simulink model "Autopilot_q_full_5may_new1"  (R2020a)
settings: Solver=ode4  StartTime=0.0  StopTime=300  FixedStep=0.01  RelTol=1e-3
undefined symbols (not defined in the file or in its folder): Aero_cofficients, Atmosphere_pert, Atmospheric_model, Counter_sensor_model, Earth, error_global, flags_global, Guidance_Flags_global, INT_global, param_guidance, Payload_data, Plane_state_mode_finish_catcher_ftr_mode, Plane_state_mode_finish_catcher_fw_mode, Plane_state_mode_finish_catcher_q_mode, Plane_state_mode_finish_catcher_rtr_mode, Plane_state_store, propulsion_model, propulsion_model_int, Structural_data, Thrust_data_store, time_global, WGS84, Wind_data, Wind_model_int, Wind_pert_factor
libraries: simulink x33, aerolibactuator x15, cstblocks x3, aerolibatmos2 x2, aerolibfltsims x1, aerolibtransform2 x1, shared6dof x1
(part 10 of 10)

== matlab function Autopilot_q_full_5may_new1/AUTOPILOT /Autopilot Transition mode/Reverse transition/Pitch Controller/theta controller/MATLAB Function3 ==
  data: t input; TT input; mass input; a_x_d input; theta_d output; data input
function theta_d  = fcn(t, TT, mass, a_x_d, data)
TT=sum(TT);
if (abs(TT)<1)
    TT=1;
end


while (abs(mass*a_x_d/TT)) >= 0.7 %% 45 deg max
    TT=TT+1;
end
theta_d=asin(-(mass/TT)*a_x_d);

if abs(theta_d)>20/57.3
    theta_d = sign(theta_d)*20.0/57.3;
end

end

== matlab function Autopilot_q_full_5may_new1/Plotter/ten_power_neg_5_zerorer/MATLAB Function ==
  data: u input; y output
function y = fcn(u)


for i=1:max(size(u))
    
    if (abs(u(i))<=0.000005)
        u(i)=0.0;
    end
    
end
y = u;

== matlab function Autopilot_q_full_5may_new1/Plotter/ten_power_neg_5_zerorer1/MATLAB Function ==
  data: u input; y output
function y = fcn(u)


for i=1:max(size(u))
    
    if (abs(u(i))<=0.000005)
        u(i)=0.0;
    end
    
end
y = u;

== matlab function Autopilot_q_full_5may_new1/Plotter/ten_power_neg_5_zerorer2/MATLAB Function ==
  data: u input; y output
function y = fcn(u)


for i=1:max(size(u))
    
    if (abs(u(i))<=0.000005)
        u(i)=0.0;
    end
    
end
y = u;

== matlab function Autopilot_q_full_5may_new1/Plotter/ten_power_neg_5_zerorer3/MATLAB Function ==
  data: u input; y output
function y = fcn(u)


for i=1:max(size(u))
    
    if (abs(u(i))<=0.0005)
        u(i)=0.0;
    end
    
end
y = u;

== matlab function Autopilot_q_full_5may_new1/Plotter/thrust to rpm/MATLAB Function ==
  data: motor_para input; u input; omega output; density input
function omega = fcn(motor_para, u,density)

b1=motor_para(1)*(density/1.225);
%d1=motor_para(2)*(density/1.225);

omega=(60.0/2*pi)*(sqrt(u/b1));


end

== matlab function Autopilot_q_full_5may_new1/Payload force and moment/Changing Mass/MATLAB Function ==
  data: ideal_Plane_state input; mass output
function mass = fcn(ideal_Plane_state)

Z=ideal_Plane_state(12);

if Z > 0.01
    
    Z=0.0;
    
end
if Z<-100
    Z=-100;
end
Z=abs(Z);
Z=0.0;
mass = 5 + 0.2*Z;
mass=5.0;
end

== matlab function Autopilot_q_full_5may_new1/Payload force and moment/MATLAB Function ==
  data: ideal_Plane_state input; Wind_f_m output; Wind_ned input; propulsion_data input; atmos_data input; payload_data input
function Wind_f_m = fcn(ideal_Plane_state, Wind_ned,propulsion_data,atmos_data, payload_data)

Wind_f_m = [0;0;0;0;0;0];
%%
b1=propulsion_data(1); % b and d of vtol propellers
d1=propulsion_data(2);
%%
rho=atmos_data(4); % density


if payload_data(1)==0
    
    Wind_f_m(:,:)=0.0;
    
else
u=ideal_Plane_state(1);
v=ideal_Plane_state(2);
w=ideal_Plane_state(3);
p=ideal_Plane_state(4);
q=ideal_Plane_state(5);
r=ideal_Plane_state(6);
phi=ideal_Plane_state(7);
theta=ideal_Plane_state(8);
psi=ideal_Plane_state(9);
X=ideal_Plane_state(10);
Y=ideal_Plane_state(11);
Z=ideal_Plane_state(12);

R_v_v1=[cos(psi) sin(psi) 0; -sin(psi) cos(psi) 0; 0 0 1];
R_v1_v2=[cos(theta) 0 -sin(theta) ;0 1 0; sin(theta) 0 cos(theta)];
R_v2_b=[1 0 0;0 cos(phi) sin(phi) ;0 -sin(phi) cos(phi)];
R_v_b=R_v2_b*R_v1_v2*R_v_v1;



V_wind_bd=R_v_b*[Wind_ned(1);Wind_ned(2);Wind_ned(3)];

ppp = [u-V_wind_bd(1); v-V_wind_bd(2); w-V_wind_bd(3)];
u_r=ppp(1);
v_r=ppp(2);
w_r=ppp(3);

V=sqrt(u_r^2+v_r^2+w_r^2);



if (u_r^2+v_r^2+w_r^2)<=0.001 
    alpha=0;
else
    alpha=atan2( w_r, u_r);
end


if norm(u_r) < 10^-3  && norm(v_r) < 10^-3 && norm(w_r) < 10^-3
    beta=0;
else
    beta = asin(v_r/sqrt(u_r^2+v_r^2+w_r^2));
end



R_b_s=[cos(alpha) 0 sin(alpha) ;0 1 0; -sin(alpha) 0 cos(alpha)]; 
R_s_w=[cos(beta) sin(beta) 0; -sin(beta) cos(beta) 0; 0 0 1];
R_w_b=(R_b_s)'*(R_s_w)';




if Z>0.01 
    Z=0.0;
end
    
if Z < -100
    Z = -100;
end

D = 0.5*rho*V*V*(0.2)*0.015*abs(Z);
D=0.0;
D_b=R_w_b*[-D;0;0];

Wind_f_m(1)=D_b(1);
Wind_f_m(2)=D_b(2);
Wind_f_m(3)=D_b(3);

payload_moment = D*abs(Z)/2;

p_m=R_w_b*[0;-payload_moment;0];


Wind_f_m(4)=p_m(1);
Wind_f_m(5)=p_m(2);
Wind_f_m(6)=p_m(3);


Wind_f_m(:,:)=0.0;

end
end

== matlab function Autopilot_q_full_5may_new1/Wind_Model/MATLAB Function ==
  data: L_u input; b0 output; sigma_u input; V input; a0 output; b1 output; a1 output; b2 output
function [b0,a0,b1,a1,b2]  = fcn(  L_u,sigma_u , V)

%num = sigma_u*sqrt(2*V/L_u);
%den = [1,V/L_u];

%tf_u = tf(num,den);
%%%%%%%%%%%%%%%%%%%%%%%%%%%%%%%%%%%
%% tf = b0 + b1.s + b2.s^2 ..
%%      ---------------------
%%      a0 + a1.s + a2.s^2 ..
%%%%%%%%%%%%%%%%%%%%%%%%%%%%%%%%%%%

% laplace inverse of b0/a1.s+a0  = b.e^-at
% here a0= V/L_u; b0=sigma_u*sqrt(2*V/L_u);
%a1=1;

a0= V/L_u;

b0=sigma_u*sqrt(2*V/L_u);

a1 =1;

b2=0;
b1=0;
% num=[0,0,b0];
% den=[0,a1,a0];


end

== matlab function Autopilot_q_full_5may_new1/Wind_Model/MATLAB Function1 ==
  data: t input; Alt input; L_u output; sigma_u output; light_turbulence_50 input; moderate_turbulence_50 input; light_turbulence_600 input; moderate_turbulence_600 input; L_v output; sigma_v output; L_w output; sigma_w output
function [L_u,sigma_u,L_v,sigma_v,L_w,sigma_w] = fcn(t, Alt, light_turbulence_50,moderate_turbulence_50,light_turbulence_600,moderate_turbulence_600)

L_u = 200; L_v = 200; L_w = 50;
sigma_u = 1.06; sigma_v = 1.06; sigma_w = 0.7;
L_u_lt_50 = 200;
sigma_u_lt_50 =  1.06;

L_v_lt_50 = 200;
sigma_v_lt_50 =  1.06;

L_w_lt_50 = 50;
sigma_w_lt_50 =  0.7;

L_u_mt_50 = 200;
sigma_u_mt_50 =  2.12;

L_v_mt_50 = 200;
sigma_v_mt_50 =  2.12;

L_w_mt_50 = 50;
sigma_w_mt_50 =  1.4;


L_u_lt_600 = 533;
sigma_u_lt_600 =  1.5;

L_v_lt_600 = 533;
sigma_v_lt_600 =  1.5;

L_w_lt_600 = 533;
sigma_w_lt_600 =  1.5;

L_u_mt_600 = 533;
sigma_u_mt_600 =  3.0;

L_v_mt_600 = 533;
sigma_v_mt_600 =  3.0;

L_w_mt_600 =533;
sigma_w_mt_600 =  3.0;

 Alt = -Alt;

if Alt<=50 && light_turbulence_50 ==1
    L_u = L_u_lt_50; L_v= L_v_lt_50 ; L_w = L_w_lt_50;
    sigma_u = sigma_u_lt_50; sigma_v= sigma_v_lt_50 ; sigma_w =sigma_w_lt_50;
end

if Alt<=50 && moderate_turbulence_50 == 1
    L_u = L_u_mt_50; L_v= L_v_mt_50 ; L_w = L_w_mt_50;
    sigma_u = sigma_u_mt_50; sigma_v= sigma_v_mt_50 ; sigma_w = sigma_w_mt_50;    
end

if Alt>=600 && light_turbulence_600 ==1  
    L_u = L_u_lt_600; L_v= L_v_lt_600 ; L_w = L_w_lt_600;
    sigma_u = sigma_u_lt_600; sigma_v= sigma_v_lt_600 ; sigma_w =sigma_w_lt_600;
end

if Alt>=600 && moderate_turbulence_600 == 1
    L_u = L_u_mt_600; L_v= L_v_mt_600 ; L_w = L_w_mt_600;
    sigma_u = sigma_u_mt_600; sigma_v= sigma_v_mt_600 ; sigma_w = sigma_w_mt_600;    
end

if Alt>50 && Alt<600 && light_turbulence_50 ==1 && light_turbulence_600 ==1
    L_u = (((L_u_lt_600 - L_u_lt_50)/(600-50))*(Alt-50)) + L_u_lt_50;
    L_v=L_u;
    L_w = (((L_w_lt_600 - L_w_lt_50)/(600-50))*(Alt-50)) + L_w_lt_50;
    
    sigma_u = (((sigma_u_lt_600 - sigma_u_lt_50)/(600-50))*(Alt-50)) + sigma_u_lt_50;
    sigma_v = sigma_u;
    sigma_w = (((sigma_w_lt_600 - sigma_w_lt_50)/(600-50))*(Alt-50)) + sigma_w_lt_50;
end

if Alt>50 && Alt<600 && moderate_turbulence_50 ==1 && moderate_turbulence_600 ==1
    L_u = (((L_u_mt_600 - L_u_mt_50)/(600-50))*(Alt-50)) + L_u_mt_50;
    L_v=L_u;
    L_w = (((L_w_mt_600 - L_w_mt_50)/(600-50))*(Alt-50)) + L_w_mt_50;
    
    sigma_u = (((sigma_u_mt_600 - sigma_u_mt_50)/(600-50))*(Alt-50)) + sigma_u_mt_50;
    sigma_v = sigma_u;
    sigma_w = (((sigma_w_mt_600 - sigma_w_mt_50)/(600-50))*(Alt-50)) + sigma_w_mt_50; 
end

if Alt>50 && Alt<600 && light_turbulence_50 ==1 && moderate_turbulence_600 ==1  
    L_u = (((L_u_mt_600 - L_u_lt_50)/(600-50))*(Alt-50)) + L_u_lt_50;
    L_v=L_u;
    L_w = (((L_w_mt_600 - L_w_lt_50)/(600-50))*(Alt-50)) + L_w_lt_50;
    
    sigma_u = (((sigma_u_mt_600 - sigma_u_lt_50)/(600-50))*(Alt-50)) + sigma_u_lt_50;
    sigma_v = sigma_u;
    sigma_w = (((sigma_w_mt_600 - sigma_w_lt_50)/(600-50))*(Alt-50)) + sigma_w_lt_50;  
end

if Alt>50 && Alt<600 && moderate_turbulence_50 ==1 && light_turbulence_600 ==1
    L_u = (((L_u_lt_600 - L_u_mt_50)/(600-50))*(Alt-50)) + L_u_mt_50;
    L_v=L_u;
    L_w = (((L_w_lt_600 - L_w_mt_50)/(600-50))*(Alt-50)) + L_w_mt_50;
    
    sigma_u = (((sigma_u_lt_600 - sigma_u_mt_50)/(600-50))*(Alt-50)) + sigma_u_mt_50;
    sigma_v = sigma_u;
    sigma_w = (((sigma_w_lt_600 - sigma_w_mt_50)/(600-50))*(Alt-50)) + sigma_w_mt_50; 
end




end

== matlab function Autopilot_q_full_5may_new1/Wind_Model/MATLAB Function2 ==
  data: L_v input; b0 output; sigma_v input; V input; a0 output; b1 output; a1 output; b2 output
function [b0,a0,b1,a1,b2] = fcn( L_v , sigma_v, V)
% 
% num = sigma_v*sqrt(3*V/L_v)*[1,V/(L_v*sqrt(3))];
% den = [1,2*V/L_v, (V/L_v)^2];

%tf_u = tf(num,den);
%%%%%%%%%%%%%%%%%%%%%%%%%%%%%%%%%%%
%% tf = b0 + b1.s + b2.s^2 ..
%%      ---------------------
%%      a0 + a1.s + a2.s^2 ..
%%%%%%%%%%%%%%%%%%%%%%%%%%%%%%%%%%%


b0 = sigma_v*sqrt(3*V/L_v)*V/(L_v*sqrt(3));
b1 = sigma_v*sqrt(3*V/L_v);
b2=0;

a0 = (V/L_v)^2;
a1 = 2*V/L_v;


% num=[b1,b0]; %% do not change size of num,den
% den=[a2,a1,a0];
end

== matlab function Autopilot_q_full_5may_new1/Wind_Model/MATLAB Function3 ==
  data: L_w input; b0 output; sigma_w input; V input; a0 output; b1 output; a1 output; b2 output
function [b0,a0,b1,a1,b2] = fcn( L_w, sigma_w , V)

% num = sigma_w*sqrt(3*V/L_w)*[1,V/(L_w*sqrt(3))];
% den = [1,2*V/L_w, (V/L_w)^2];
%tf_u = tf(num,den);
%%%%%%%%%%%%%%%%%%%%%%%%%%%%%%%%%%%
%% tf = b0 + b1.s + b2.s^2 ..
%%      ---------------------
%%      a0 + a1.s + a2.s^2 ..
%%%%%%%%%%%%%%%%%%%%%%%%%%%%%%%%%%%


b0 = sigma_w*sqrt(3*V/L_w)*V/(L_w*sqrt(3));
b1 = sigma_w*sqrt(3*V/L_w);
b2 = 0;

a0 = (V/L_w)^2;
a1 = 2*V/L_w;


% num=[b1,b0]; %% do not change size of num,den
% den=[a2,a1,a0];

end

== matlab function Autopilot_q_full_5may_new1/Wind_Model/System3/Subsystem1/MATLAB Function ==
  data: i input; ii input; num input; den input; y input; yyy output; yy input

function yyy = fcn(i, ii, num,den,y, yy)
%#codegen

b0= num(2);
b1= num(1);

a0=den(3);
a1=den(2);
a2=den(1); 

yyy  = (b0*i + b1*ii -yy*a1 - y*a0)/a2;

== matlab function Autopilot_q_full_5may_new1/Wind_Model/System3/Subsystem4/MATLAB Function ==
  data: i input; num input; den input; y input; yy output
function yy = fcn(i,num,den,y)
%#codegen

b0= num(1);
a0=den(2);
a1=den(1);
                                                                                                                                                                                                                                                                                                                                                                                                                                                                                                                                                                                                            
yy= (b0*i-y*a0)/a1;

== matlab function Autopilot_q_full_5may_new1/Wind_Model/System3/Subsystem5/MATLAB Function ==
  data: i input; ii input; num input; den input; y input; yyy output; yy input

function yyy = fcn(i,ii, num,den,y, yy)
%#codegen

b0= num(2);
b1= num(1);

a0=den(3);
a1=den(2);
a2=den(1); 

yyy  = (b0*i + b1*ii -yy*a1 - y*a0)/a2;

== matlab function Autopilot_q_full_5may_new1/Wind_Model/Wind Speed ==
  data: Euler_angle input; V_ned input; V output; u output; v output; w output
function [V,u,v,w] = fcn(Euler_angle, V_ned)

phi=Euler_angle(1);
theta=Euler_angle(2);
psi=Euler_angle(3);


R_v_v1=[cos(psi) sin(psi) 0; -sin(psi) cos(psi) 0; 0 0 1];
R_v1_v2=[cos(theta) 0 -sin(theta) ;0 1 0; sin(theta) 0 cos(theta)];
R_v2_b=[1 0 0;0 cos(phi) sin(phi) ;0 -sin(phi) cos(phi)];
R_v_b=R_v2_b*R_v1_v2*R_v_v1;



V_bd=R_v_b*[ V_ned(1);  V_ned(2);  V_ned(3)];


V = norm(V_ned);
u=V_bd(1);
v=V_bd(2);
w=V_bd(3);


end

== matlab function Autopilot_q_full_5may_new1/Wind_Model/System3/Wind Speed ==
  data: uu input; V output; u output; v output; w output
function [V,u,v,w] = fcn(uu)

u1=uu(1);
u2=uu(2);
u3=uu(3);
u=u1;
v=u2;
w=u3;
V=sqrt(u1*u1 + u2*u2 + u3*u3);
end

== matlab function Autopilot_q_full_5may_new1/Wind_Model/Wind Speed1 ==
  data: Euler_angle input; V_bd input; V_ned output
function V_ned  = fcn(Euler_angle, V_bd)

phi=Euler_angle(1);
theta=Euler_angle(2);
psi=Euler_angle(3);


R_v_v1=[cos(psi) sin(psi) 0; -sin(psi) cos(psi) 0; 0 0 1];
R_v1_v2=[cos(theta) 0 -sin(theta) ;0 1 0; sin(theta) 0 cos(theta)];
R_v2_b=[1 0 0;0 cos(phi) sin(phi) ;0 -sin(phi) cos(phi)];
R_v_b=R_v2_b*R_v1_v2*R_v_v1;



V_ned=R_v_b'*[ V_bd(1);  V_bd(2);  V_bd(3)];





end

== matlab function Autopilot_q_full_5may_new1/All SENSOR MODEL2/INS BODY RATES/MATLAB Function2 ==
  data: count_temp output; t input; count output; frequency_plant input; y output size=[1,3]; frequency_imu input; frequency_nav input; in input; in_old input; count input; count_temp input
function [count_temp,count,y] = fcn(t, frequency_plant,frequency_imu,frequency_nav, in, in_old, count,count_temp)
%#codegen

%step_size=floor(frequecy_plant/frequecy_nav);

step_size = 1/frequency_imu;
y= zeros(1,3);
if rem(t,step_size) ==0 && (count_temp==1)
    y(1)=in(1);
    y(2)=in(2);
    y(3)=in(3);
    count = count + 1;
    count_temp=0;
else
    y(1)=in_old(1);
    y(2)=in_old(2);
    y(3)=in_old(3);
    count_temp=1;
end



end

== matlab function Autopilot_q_full_5may_new1/All SENSOR MODEL2/INS EULER ANGLE/MATLAB Function2 ==
  data: count_temp output; t input; count output; frequency_plant input; y output size=[1,3]; frequency_imu input; frequency_nav input; in input; in_old input; count input; count_temp input
function [count_temp,count,y] = fcn(t, frequency_plant,frequency_imu,frequency_nav, in, in_old, count,count_temp)
%#codegen

%step_size=floor(frequecy_plant/frequecy_nav);

step_size = 1/frequency_nav;
y= zeros(1,3);
if rem(t,step_size) ==0 && (count_temp==1)
    y(1)=in(1);
    y(2)=in(2);
    y(3)=in(3);
    count = count + 1;
    count_temp=0;
else
    y(1)=in_old(1);
    y(2)=in_old(2);
    y(3)=in_old(3);
    count_temp=1;
end



end

== matlab function Autopilot_q_full_5may_new1/All SENSOR MODEL2/INS NAV POSITION/MATLAB Function2 ==
  data: count_temp output; t input; count output; frequency_plant input; y output size=[1,3]; frequency_imu input; frequency_nav input; in input; in_old input; count input; count_temp input
function [count_temp,count,y] = fcn(t, frequency_plant,frequency_imu,frequency_nav, in, in_old, count,count_temp)
%#codegen

%step_size=floor(frequecy_plant/frequecy_nav);

step_size = 1/frequency_nav;
y= zeros(1,3);
if rem(t,step_size) ==0 && (count_temp==1)
    y(1)=in(1);
    y(2)=in(2);
    y(3)=in(3);
    count = count + 1;
    count_temp=0;
else
    y(1)=in_old(1);
    y(2)=in_old(2);
    y(3)=in_old(3);
    count_temp=1;
end



end

== matlab function Autopilot_q_full_5may_new1/All SENSOR MODEL2/INS NAV VELOCITY  /MATLAB Function2 ==
  data: count_temp output; t input; count output; frequency_plant input; y output size=[1,3]; frequency_imu input; frequency_nav input; in input; in_old input; count input; count_temp input
function [count_temp,count,y] = fcn(t, frequency_plant,frequency_imu,frequency_nav, in, in_old, count,count_temp)
%#codegen

%step_size=floor(frequecy_plant/frequecy_nav);

step_size = 1/frequency_nav;
y= zeros(1,3);
if rem(t,step_size) ==0 && (count_temp==1)
    y(1)=in(1);
    y(2)=in(2);
    y(3)=in(3);
    count = count + 1;
    count_temp=0;
else
    y(1)=in_old(1);
    y(2)=in_old(2);
    y(3)=in_old(3);
    count_temp=1;
end



end

== matlab function Autopilot_q_full_5may_new1/All SENSOR MODEL2/MATLAB Function ==
  settings: updateMethod=DISCRETE
  data: sigma input; mu input; y output
function y = fcn(sigma,mu)
y=normrnd(mu,sigma);
end
